simulink model "part2"  (R2020a)
settings: Solver=FixedStepAuto  StartTime=0.0  StopTime=150  FixedStep=0.1  RelTol=1e-3
values from neighbouring files (symbols this model uses):
  A = [zeros(3), eye(3) ... (first row only)    [initEKF.m]    (also in initEKF.mat = [0 0 0 -0.394784176044 0 0 0 0 0 0 -0.394784176044 0 ... (36)
  B = [0 0 0 0 0 0 1.46677031844e-07 0 0 0 0 0 ... (27 elements, 9x3)]    [ExtendedKalmanFilter.mat]    (also in initEKF.m = [zeros(6,3); initEKF.mat = [0 0 0 0 0 0 0 0 0 0 0 0 ... (45 elements, 15x3)]; initObserverInput.m = [zeros(6,3);zeros(3,3);zeros(3,3);invM]; initObserverInput.mat = [0 0 0 0 0 0 0 0 0 0 0 0 ... (45 elements, 15x3)])
  ConstSPSuge = 0    [ExtendedKalmanFilter.mat]    (also in doSimPart2.m; init.m; init1.m; init_weather.m)
  ConstSPSway = 0    [ExtendedKalmanFilter.mat]    (also in doSimPart2.m; init.m; init1.m; init_weather.m)
  ConstSPYaw = 0    [ExtendedKalmanFilter.mat]    (also in doSimPart2.m; init.m; init1.m; init_weather.m)
  Curent_Slaw_var = 0    [ExtendedKalmanFilter.mat]    (also in doSimPart2.m; init.m; init1.m; init_weather.m = 1)
  Current_Head_mu = 0.001    [ExtendedKalmanFilter.mat]    (also in doSimPart2.m; init.m; init1.m; init_weather.m)
  Current_Head_Sample_time = 1    [ExtendedKalmanFilter.mat]    (also in doSimPart2.m; init.m; init1.m; init_weather.m)
  Current_input_type = 0    [ExtendedKalmanFilter.mat]    (also in doSimPart2.m; init.m; init1.m; init_weather.m)
  Current_Speed = 0    [ExtendedKalmanFilter.mat]    (also in doSimPart2.m = 0.2; init.m; init1.m; init_weather.m = 0.2)
  CurrHead =     [ExtendedKalmanFilter.mat]
  D = [264860  0  0; 0  881640  0; 0  0  337740000]    [ExtendedKalmanFilter.mat]    (also in initEKF.m = [2.6486e5, 0, 0; initEKF.mat; initObserverInput.m = diag([2.6486e5, 8.8164e5, 3.3774e8]); initObserverInput.mat)
  E = [0 0 0 1 0 0 0 0 0 0 0 0 ... (27 elements, 9x3)]    [ExtendedKalmanFilter.mat]    (also in initEKF.m = [Ew, zeros(6,3); initEKF.mat = [0 0 0 0.01 0 0 0 0 0 0 0 0 ... (90 elements, 15x6)]; initObserverInput.m = [Ew, zeros(6,3); zeros(3), zeros(3); zeros(3), Eb; zeros(3),; initObserverInput.mat = [0 0 0 0.01 0 0 0 0 0 0 0 0 ... (90 elements, 15x6)])
  H = [1 0 0 0 1 0 0 0 1 0 0 0 ... (27 elements, 3x9)]    [ExtendedKalmanFilter.mat]    (also in initEKF.m = [C, eye(3), zeros(3), zeros(3)]; initEKF.mat = [0 0 0 0 0 0 0 0 0 1 0 0 ... (45 elements, 3x15)]; initObserverInput.m = [Cw, eye(3), zeros(3), zeros(3)]; initObserverInput.mat = [0 0 0 0 0 0 0 0 0 1 0 0 ... (45 elements, 3x15)])
  h = polar(Wind_Headind_EF.Data(:,1),Wind_Speed.Data(:,1))    [init.m]    (also in init1.m; initEKF.m = 0.1; initEKF.mat = 0.1; initObserverInput.m = 0.1)
  invM = inv(M)    [initEKF.m]    (also in initEKF.mat = [1.46677031844e-07  0  0; 0  1.2695973473e-07  9.23036390732; initObserverInput.m; initObserverInput.mat = [1.46677031844e-07  0  0; 0  1.2695973473e-07  9.23036390732)
  invT = inv(T)    [initEKF.m]    (also in initEKF.mat = [0.001  0  0; 0  0.001  0; 0  0  0.001])
  Kd_surge = 1868784.40925    [ExtendedKalmanFilter.mat]    (also in doSimPart2.m = 2*0.7*sqrt(6.4794^5+6.362*10^6)*sqrt(Kp_surge); init.m = 2*0.7*sqrt(6.4794^5+6.362*10^6)*sqrt(Kp_surge); init1.m = 2*0.7*sqrt(6.4794^5+6.362*10^6)*sqrt(Kp_surge); init_weather.m = 2*0.7*sqrt(6.4794^5+6.362*10^6)*sqrt(Kp_surge))
  Kd_sway = 3746851.89423    [ExtendedKalmanFilter.mat]    (also in doSimPart2.m = 2*0.7*sqrt(2.157*10^6+6.362*10^6)*sqrt(Kp_sway); init.m = 2*0.7*sqrt(2.157*10^6+6.362*10^6)*sqrt(Kp_sway); init1.m = 2*0.7*sqrt(2.157*10^6+6.362*10^6)*sqrt(Kp_sway); init_weather.m = 2*0.7*sqrt(2.157*10^6+6.362*10^6)*sqrt(Kp_sway))
  Kd_yaw = 3338344318.3    [ExtendedKalmanFilter.mat]    (also in doSimPart2.m = 2*0.7*sqrt(1.0711*10^9+2.724*10^9)*sqrt(Kp_yaw); init.m = 2*0.7*sqrt(1.0711*10^9+2.724*10^9)*sqrt(Kp_yaw); init1.m = 2*0.7*sqrt(1.0711*10^9+2.724*10^9)*sqrt(Kp_yaw); init_weather.m = 2*0.7*sqrt(1.0711*10^9+2.724*10^9)*sqrt(Kp_yaw))
  Ki_surge = 18000    [ExtendedKalmanFilter.mat]    (also in doSimPart2.m; init.m; init1.m; init_weather.m)
  Ki_sway = 80000    [ExtendedKalmanFilter.mat]    (also in doSimPart2.m; init.m; init1.m; init_weather.m)
  Ki_yaw = 150000000    [ExtendedKalmanFilter.mat]    (also in doSimPart2.m; init.m; init1.m; init_weather.m = 150000)
  Kp_surge = 279569.493868    [ExtendedKalmanFilter.mat]    (also in doSimPart2.m; init.m; init1.m; init_weather.m = 195698.645708)
  Kp_sway = 840791.598929    [ExtendedKalmanFilter.mat]    (also in doSimPart2.m; init.m; init1.m; init_weather.m = 588554.11925)
  Kp_yaw = 1498245426.5    [ExtendedKalmanFilter.mat]    (also in doSimPart2.m; init.m; init1.m; init_weather.m = 104877179.855)
  p_bar = zeros(15)    [initEKF.m]    (also in initEKF.mat = [0 0 0 0 0 0 0 0 0 0 0 0 ... (225 elements, 15x15)])
  Q = [1000000000000  0  0; 0  1000000000000  0; 0  0  100000000000000]    [ExtendedKalmanFilter.mat]    (also in initEKF.m = [10^4, 0, 0, 0, 0, 0; initEKF.mat = [10000 0 0 0 0 0 0 10000 0 0 0 0 ... (36 elements, 6x6)]; initObserverInput.m = diag([ 10^4 10^4 10^3 10^9 10^9 10^9]); initObserverInput.mat = [10000 0 0 0 0 0 0 10000 0 0 0 0 ... (36 elements, 6x6)])
  R = [1.15e-05  0  0; 0  1.2e-06  0; 0  0  4e-08]    [ExtendedKalmanFilter.mat]    (also in initEKF.m = [1, 0,0; initEKF.mat = [1  0  0; 0  1  0; 0  0  0.1]; initObserverInput.m = diag([1,1,0.1]); initObserverInput.mat = [1  0  0; 0  1  0; 0  0  0.1])
  thrusters =     [ExtendedKalmanFilter.mat]
  typeOfSimulation = 2    [ExtendedKalmanFilter.mat]    (also in doSimPart2.m = 0; init.m; init1.m; init_weather.m)
  vessel =     [ExtendedKalmanFilter.mat]
  Wind_gust_k = 0.0026    [ExtendedKalmanFilter.mat]    (also in doSimPart2.m; init.m; init1.m; init_weather.m)
  Wind_gust_L = 1800    [ExtendedKalmanFilter.mat]    (also in doSimPart2.m; init.m; init1.m; init_weather.m)
  Wind_gust_nfreq = 1000    [ExtendedKalmanFilter.mat]    (also in doSimPart2.m; init.m; init1.m; init_weather.m)
  Wind_gust_phi = [1.94720348827 2.24175439974 2.07841268688 2.94269508899 2.5189968857 3.92559282604 1.02965824361 5.79326836705 3.39416152385 6.24100933894 1.9296881265 4.15801677987 ... (1000 elements, 1000x1)]    [ExtendedKalmanFilter.mat]    (also in doSimPart2.m = 2*pi * rand(Wind_gust_nfreq,1); init.m = 2*pi * rand(Wind_gust_nfreq,1); init1.m = 2*pi * rand(Wind_gust_nfreq,1); init_weather.m = 2*pi * rand(Wind_gust_nfreq,1))
  Wind_Gust_type = 0    [ExtendedKalmanFilter.mat]    (also in doSimPart2.m = 1; init.m; init1.m; init_weather.m = 1)
  Wind_Head_mean = 1.57079632679    [ExtendedKalmanFilter.mat]    (also in doSimPart2.m = vector_Headings_rad; init.m; init1.m; init_weather.m = 0)
  Wind_Head_mu = 0.001    [ExtendedKalmanFilter.mat]    (also in doSimPart2.m; init.m; init1.m; init_weather.m)
  Wind_Head_Sample_time = 1    [ExtendedKalmanFilter.mat]    (also in doSimPart2.m; init.m; init1.m; init_weather.m)
  Wind_Heading_type = 0    [ExtendedKalmanFilter.mat]    (also in doSimPart2.m; init.m; init1.m; init_weather.m = 1)
  Wind_U10 = 0    [ExtendedKalmanFilter.mat]    (also in doSimPart2.m = 15; init.m; init1.m; init_weather.m)
  Wind_U_mean = 0    [ExtendedKalmanFilter.mat]    (also in doSimPart2.m = Umean; init.m = Umean; init1.m = Umean; init_weather.m = Umean)
  Wind_U_mu = 0.001    [ExtendedKalmanFilter.mat]    (also in doSimPart2.m; init.m; init1.m; init_weather.m)
  Wind_U_Sample_time = 1    [ExtendedKalmanFilter.mat]    (also in doSimPart2.m; init.m; init1.m; init_weather.m)
  Wind_U_type = 0    [ExtendedKalmanFilter.mat]    (also in doSimPart2.m = 1; init.m; init1.m; init_weather.m = 1)
  x_bar = zeros(15,1)    [initEKF.m]    (also in initEKF.mat = [0 0 0 0 0 0 0 0 0 0 0 0 ... (15 elements, 15x1)])
undefined symbols (not defined in the file or in its folder): Hoerner
libraries: marine_gnc x10, simulink x4, marine_hydro x2
(part 1 of 2)
settings Model: Creator=jonbjor  LastModifiedBy=maria
settings DataIOCC: ReturnWorkspaceOutputs=off
settings DebuggingCC: ArithmeticOperatorsInVariantConditions=warning
settings SFSimCC: SimUseLocalCustomCode=off  CustomCodeUndefinedFunction=UseInterfaceOnly
settings RTWCC: RTWUseLocalCustomCode=off

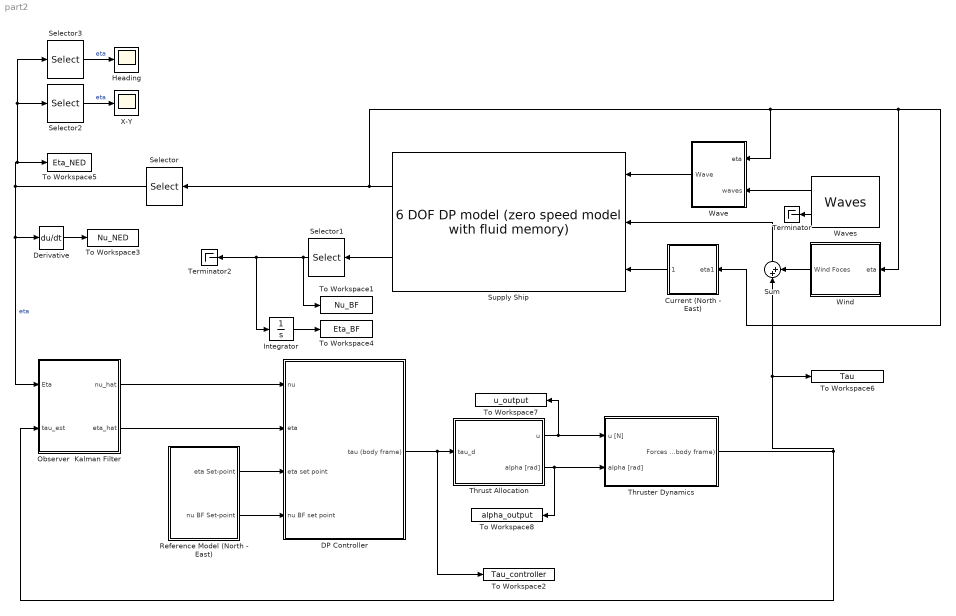
== system part2 ==
  Current (North - East) : Subsystem
  DP Controller : Subsystem
  Derivative : Derivative
  Heading : Scope
  Integrator : Integrator
  Observer  Kalman Filter : Subsystem
  Reference Model (North - East) : Subsystem
  Selector : Selector  InputPortWidth=6  IndexOptions=Index vector (dialog)  Indices=[1 2 6]  OutputSizes=1
  Selector1 : Selector  InputPortWidth=6  IndexOptions=Index vector (dialog)  Indices=[1 2 6]  OutputSizes=1
  Selector2 : Selector  InputPortWidth=3  IndexOptions=Index vector (dialog)  Indices=[1 2]  OutputSizes=1
  Selector3 : Selector  InputPortWidth=3  IndexOptions=Index vector (dialog)  Indices=3  OutputSizes=1
  Sum : Sum  Inputs=|++
  Supply Ship : marine_hydro/Hydro Library/6 DOF DP model  (zero speed model with fluid memory)  ABC=vesselABC  rho=1025  Axc=0.9*vessel.main.T*vessel.main.B  Ayc=0.9*vessel.main.T*vessel.main.Lpp  CX=1  CY_2D=Hoerner(vessel.main.B,vessel.main.T)  Bv=vessel.Bv  mask(6 DOF zero speed model){}
      link override "Integrator1 ": InitialCondition=nu0
      link override Integrator2: InitialCondition=eta0
      settings: SourceProductName=MSS Hydro
      mask Display:
      | image('supply.jpg');
      | color('white'); port_label('output', 1, 'eta')
      | color('white'); port_label('output', 2, 'nu')
      | color('white'); port_label('input', 1, 'tau_wave')
      | color('white'); port_label('input', 2, 'tau')
      | color('white'); port_label('input', 3, 'nu_c')
  Terminator : Terminator
  Terminator2 : Terminator
  Thrust Allocation : Subsystem
  Thruster Dynamics : Subsystem  mask{thrusterfault=off}
      mask prompts: thrusterfault "Fault on thruster #2 and #5?"
  To Workspace1 : ToWorkspace  VariableName=Nu_BF  SaveFormat=Timeseries  SampleTime=-1
  To Workspace2 : ToWorkspace  VariableName=Tau_controller  SaveFormat=Timeseries  SampleTime=-1
  To Workspace3 : ToWorkspace  VariableName=Nu_NED  SaveFormat=Timeseries  SampleTime=-1
  To Workspace4 : ToWorkspace  VariableName=Eta_BF  SaveFormat=Timeseries  SampleTime=-1
  To Workspace5 : ToWorkspace  VariableName=Eta_NED  SaveFormat=Timeseries  SampleTime=-1
  To Workspace6 : ToWorkspace  VariableName=Tau  SaveFormat=Timeseries  SampleTime=-1
  To Workspace7 : ToWorkspace  VariableName=u_output  SaveFormat=Timeseries  SampleTime=-1
  To Workspace8 : ToWorkspace  VariableName=alpha_output  SaveFormat=Timeseries  SampleTime=-1
  Wave : Subsystem  mask{waveforces=on}
      mask prompts: waveforces "Waveforces enabled"
  Waves : marine_gnc/Environment/Waves/Waves  spectrum_type=ITTC  disp_flag=on  plot_spectrum=off  plot_realization=off  hs=Significant_wave_height_Hs  omega_peak=Peak_frequency_omega_0  psi_mean=Mean_wave_direction  gamma=-1  spread=2  depth=inf  nfreq=20  ndir=10  energylim=0.005  freq_cutoff=3  dir_cutoff=0  rand_seed=123  rand_freq=on  rand_dir=on  Zeta_a=0  Omega=0  Phase=0  Wavenum=0  Psi=0
      settings: SourceProductName=MSS GNC
  Wind : Subsystem
  X-Y : Scope
  wires:
  Supply Ship/2 -> Selector1/1
  Reference Model (North - East)/1(eta Set-point) -> DP Controller/3(eta set point)
  Supply Ship/1 -> Current (North - East)/1(eta1), Wind/1(eta), Wave/1(eta), Selector/1
  Waves/1 -> Wave/2(waves)
  Waves/2 -> Terminator/1
  Sum/1 -> Supply Ship/2
  Thrust Allocation/2(alpha [rad]) -> Thruster Dynamics/2(alpha [rad]), To Workspace8/1
  Current (North - East)/1(Current) -> Supply Ship/3
  Selector/1 -> Observer  Kalman Filter/1(Eta), Derivative/1, Selector3/1, Selector2/1, To Workspace5/1  "eta"
  Wind/1(Wind Foces) -> Sum/2
  Derivative/1 -> To Workspace3/1
  Integrator/1 -> To Workspace4/1
  Wave/1(Wave) -> Supply Ship/1
  Reference Model (North - East)/2(nu BF Set-point) -> DP Controller/4(nu BF set point)
  Thrust Allocation/1(u) -> Thruster Dynamics/1(u [N]), To Workspace7/1
  Selector1/1 -> To Workspace1/1, Terminator2/1, Integrator/1
  Observer  Kalman Filter/1(nu_hat) -> DP Controller/1(nu)
  Observer  Kalman Filter/2(eta_hat) -> DP Controller/2(eta)
  Selector2/1 -> X-Y/1  "eta"
  Selector3/1 -> Heading/1  "eta"
  DP Controller/1(tau (body frame)) -> To Workspace2/1, Thrust Allocation/1(tau_d)
  Thruster Dynamics/1("Forces (body frame) ") -> Observer  Kalman Filter/2(tau_est), Sum/1, To Workspace6/1

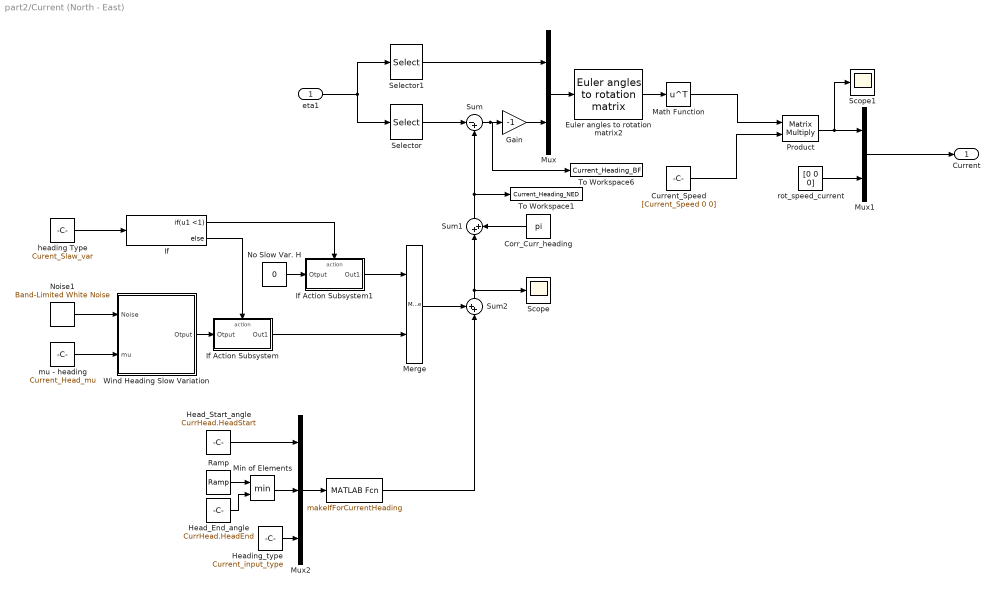
== system part2/Current (North - East) ==
  eta1 : Inport
  " " : MATLABFcn  MATLABFcn=makeIfForCurrentHeading
  Corr_Curr_heading : Constant  Value=pi
  Current_Speed : Constant  Value=[Current_Speed 0 0]
  Euler angles to rotation matrix2 : marine_gnc/Models/ Kinematics/Euler angles to rotation matrix
      settings: SourceProductName=MSS GNC
  Gain : Gain  Gain=-1
  Head_End_angle : Constant  Value=CurrHead.HeadEnd
  Head_Start_angle : Constant  Value=CurrHead.HeadStart
  Heading_type : Constant  Value=Current_input_type
  If : If  IfExpression=u1 <1
  If Action Subsystem : Subsystem  TreatAsAtomicUnit=on
  If Action Subsystem1 : Subsystem  TreatAsAtomicUnit=on
  Math Function : Math  Operator=transpose  SaturateOnIntegerOverflow=on
  Merge : Merge
  Min of Elements : MinMax  Inputs=2
  Mux : Mux  Inputs=2
  Mux1 : Mux  Inputs=2
  Mux2 : Mux  Inputs=3
  No Slow Var. H : Constant  Value=0
  Noise1 : simulink/Sources/Band-Limited White Noise  Cov=Current_Head_noise_power  Ts=Current_Head_Sample_time  seed=Current_Head_Seed
  Product : Product  Inputs=**  Multiplication=Matrix(*)  SaturateOnIntegerOverflow=on  OutDataTypeStr=Inherit: Same as first input
  Ramp : simulink/Sources/Ramp  slope=CurrHead.Slope  start=CurrHead.TimeStart  InitialOutput=CurrHead.HeadStart
  Scope : Scope
  Scope1 : Scope
  Selector : Selector  InputPortWidth=6  IndexOptions=Index vector (dialog)  Indices=[6]  OutputSizes=1
  Selector1 : Selector  InputPortWidth=6  IndexOptions=Index vector (dialog)  Indices=[4 5]  OutputSizes=1
  Sum : Sum  Inputs=|-+
  Sum1 : Sum  Inputs=|++
  Sum2 : Sum  Inputs=++|
  To Workspace1 : ToWorkspace  VariableName=Current_Heading_NED  SaveFormat=Timeseries  SampleTime=-1
  To Workspace6 : ToWorkspace  VariableName=Current_Heading_BF  SaveFormat=Timeseries  SampleTime=-1
  Wind Heading Slow Variation : Subsystem
  heading Type : Constant  Value=Curent_Slaw_var
  mu - heading : Constant  Value=Current_Head_mu
  rot_speed_current : Constant  Value=[0 0 0]
  Current : Outport  VectorParamsAs1DForOutWhenUnconnected=off
  wires:
  Sum2/1 -> Scope/1, Sum1/1
  eta1/1 -> Selector/1, Selector1/1
  Merge/1 -> Sum2/1
  mu - heading/1 -> Wind Heading Slow Variation/2(mu)
  " "/1 -> Sum2/2
  If Action Subsystem1/1(Out1) -> Merge/1
  Sum1/1 -> To Workspace1/1, Sum/2
  If Action Subsystem/1(Out1) -> Merge/2
  Wind Heading Slow Variation/1(Otput) -> If Action Subsystem/1(Otput)
  No Slow Var. H/1 -> If Action Subsystem1/1(Otput)
  If/2 -> If Action Subsystem/Action
  Selector1/1 -> Mux/1
  If/1 -> If Action Subsystem1/Action
  Selector/1 -> Sum/1
  Mux/1 -> Euler angles to rotation matrix2/1
  heading Type/1 -> If/1
  Corr_Curr_heading/1 -> Sum1/2
  Product/1 -> Scope1/1, Mux1/1
  Noise1/1 -> Wind Heading Slow Variation/1(Noise)
  Current_Speed/1 -> Product/2
  Head_Start_angle/1 -> Mux2/1
  Euler angles to rotation matrix2/1 -> Math Function/1
  rot_speed_current/1 -> Mux1/2
  Mux2/1 -> " "/1
  Mux1/1 -> Current/1
  Min of Elements/1 -> Mux2/2
  Math Function/1 -> Product/1
  Heading_type/1 -> Mux2/3
  Ramp/1 -> Min of Elements/1
  Head_End_angle/1 -> Min of Elements/2
  Sum/1 -> Gain/1, To Workspace6/1
  Gain/1 -> Mux/2

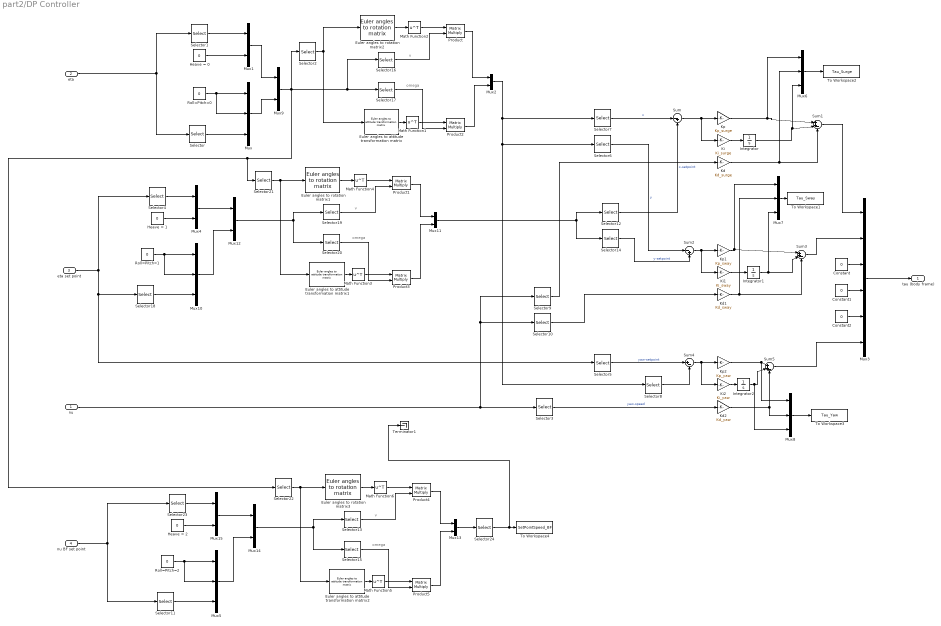
== system part2/DP Controller ==
  note: omega
  note: omega
  note: v
  note: v
  note: omega
  note: v
  nu : Inport
  eta : Inport  Port=2
  eta set point : Inport  Port=3
  nu BF set point : Inport  Port=4
  Constant : Constant  Value=0
  Constant1 : Constant  Value=0
  Constant2 : Constant  Value=0
  Euler angles to rotation matrix1 : marine_gnc/Models/ Kinematics/Euler angles to rotation matrix
      settings: SourceProductName=MSS GNC
  Euler angles to rotation matrix2 : marine_gnc/Models/ Kinematics/Euler angles to rotation matrix
      settings: SourceProductName=MSS GNC
  Euler angles to rotation matrix3 : marine_gnc/Models/ Kinematics/Euler angles to rotation matrix
      settings: SourceProductName=MSS GNC
  Euler angles to attitude transformation matrix : marine_gnc/Models/ Kinematics/Euler angles to attitude transformation matrix
      settings: SourceProductName=MSS GNC
  Euler angles to attitude transformation matrix1 : marine_gnc/Models/ Kinematics/Euler angles to attitude transformation matrix
      settings: SourceProductName=MSS GNC
  Euler angles to attitude transformation matrix2 : marine_gnc/Models/ Kinematics/Euler angles to attitude transformation matrix
      settings: SourceProductName=MSS GNC
  Heave = 0 : Constant  Value=0
  Heave = 1 : Constant  Value=0
  Heave = 2 : Constant  Value=0
  Integrator : Integrator
  Integrator1 : Integrator
  Integrator2 : Integrator
  Kd : Gain  Gain=Kd_surge
  Kd1 : Gain  Gain=Kd_sway
  Kd2 : Gain  Gain=Kd_yaw
  Ki : Gain  Gain=Ki_surge
  Ki1 : Gain  Gain=Ki_sway
  Ki2 : Gain  Gain=Ki_yaw
  Kp : Gain  Gain=Kp_surge
  Kp1 : Gain  Gain=Kp_sway
  Kp2 : Gain  Gain=Kp_yaw
  Math Function{1..6} (6 alike) : Math  Operator=transpose  SaturateOnIntegerOverflow=on
  Mux{,5..8,10} (6 alike) : Mux  Inputs=3
  Mux{1..2,4,9,11..15} (9 alike) : Mux  Inputs=2
  Mux3 : Mux  Inputs=6
  Product{,1..5} (6 alike) : Product  Inputs=**  Multiplication=Matrix(*)  SaturateOnIntegerOverflow=on  OutDataTypeStr=Inherit: Same as first input
  Roll=Pitch=0 : Constant  Value=0
  Roll=Pitch=1 : Constant  Value=0
  Roll=Pitch=2 : Constant  Value=0
  Selector{,5,11,18} (4 alike) : Selector  InputPortWidth=3  IndexOptions=Index vector (dialog)  Indices=[3]  OutputSizes=1
  Selector1 : Selector  InputPortWidth=3  IndexOptions=Index vector (dialog)  Indices=[1 2]  OutputSizes=1
  Selector10 : Selector  InputPortWidth=3  IndexOptions=Index vector (dialog)  Indices=2  OutputSizes=1
  Selector12 : Selector  InputPortWidth=6  IndexOptions=Index vector (dialog)  Indices=1  OutputSizes=1
  Selector13 : Selector  InputPortWidth=6  IndexOptions=Index vector (dialog)  Indices=[1 2 3]  OutputSizes=1
  Selector14 : Selector  InputPortWidth=6  IndexOptions=Index vector (dialog)  Indices=2  OutputSizes=1
  Selector{2,15,17,20..22} (6 alike) : Selector  InputPortWidth=6  IndexOptions=Index vector (dialog)  Indices=[4 5 6]  OutputSizes=1
  Selector16 : Selector  InputPortWidth=6  IndexOptions=Index vector (dialog)  Indices=[1 2 3]  OutputSizes=1
  Selector19 : Selector  InputPortWidth=6  IndexOptions=Index vector (dialog)  Indices=[1 2 3]  OutputSizes=1
  Selector23 : Selector  InputPortWidth=3  IndexOptions=Index vector (dialog)  Indices=[1 2]  OutputSizes=1
  Selector24 : Selector  InputPortWidth=6  IndexOptions=Index vector (dialog)  Indices=[1 2 6]  OutputSizes=1
  Selector3 : Selector  InputPortWidth=3  IndexOptions=Index vector (dialog)  Indices=3  OutputSizes=1
  Selector4 : Selector  InputPortWidth=3  IndexOptions=Index vector (dialog)  Indices=[1 2]  OutputSizes=1
  Selector6 : Selector  InputPortWidth=6  IndexOptions=Index vector (dialog)  Indices=2  OutputSizes=1
  Selector7 : Selector  InputPortWidth=6  IndexOptions=Index vector (dialog)  Indices=1  OutputSizes=1
  Selector8 : Selector  InputPortWidth=6  IndexOptions=Index vector (dialog)  Indices=[6]  OutputSizes=1
  Selector9 : Selector  InputPortWidth=3  IndexOptions=Index vector (dialog)  Indices=1  OutputSizes=1
  Sum : Sum  Inputs=|-+
  Sum1 : Sum  Inputs=|++-
  Sum2 : Sum  Inputs=|-+
  Sum3 : Sum  Inputs=|++-
  Sum4 : Sum  Inputs=|+-
  Sum5 : Sum  Inputs=|++-
  Terminator1 : Terminator
  To Workspace1 : ToWorkspace  VariableName=Tau_Sway  SaveFormat=Timeseries  SampleTime=-1
  To Workspace2 : ToWorkspace  VariableName=Tau_Surge  SaveFormat=Timeseries  SampleTime=-1
  To Workspace3 : ToWorkspace  VariableName=Tau_Yaw  SaveFormat=Timeseries  SampleTime=-1
  To Workspace4 : ToWorkspace  VariableName=SetPointSpeed_BF  SaveFormat=Timeseries  SampleTime=-1
  tau (body frame) : Outport  VectorParamsAs1DForOutWhenUnconnected=off
  wires:
  Selector20/1 -> Product3/2
  Mux4/1 -> Mux12/1
  Selector2/1 -> Euler angles to attitude transformation matrix/1, Euler angles to rotation matrix2/1
  Product1/1 -> Mux11/1
  Mux10/1 -> Mux12/2
  Mux8/1 -> To Workspace3/1
  Euler angles to rotation matrix1/1 -> Math Function4/1
  Product/1 -> Mux2/1
  Selector17/1 -> Product2/2
  Kp2/1 -> Mux8/1, Sum5/1
  Ki1/1 -> Integrator1/1
  Mux6/1 -> To Workspace2/1
  Euler angles to rotation matrix2/1 -> Math Function2/1
  Selector6/1 -> Sum2/1  "y"
  Selector/1 -> Mux/3
  Sum4/1 -> Ki2/1, Kp2/1
  Kp1/1 -> Mux7/1, Sum3/1
  Product2/1 -> Mux2/2
  Constant1/1 -> Mux3/4
  Selector18/1 -> Mux10/3
  Sum2/1 -> Ki1/1, Kp1/1
  eta set point/1 -> Selector4/1, Selector18/1, Selector5/1
  Kd1/1 -> Mux7/2, Sum3/3
  Mux1/1 -> Mux9/1
  Sum1/1 -> Mux3/1
  Kd2/1 -> Mux8/2, Sum5/3
  Roll=Pitch=1/1 -> Mux10/1, Mux10/2
  Ki/1 -> Integrator/1
  Product3/1 -> Mux11/2
  Selector4/1 -> Mux4/1
  Math Function4/1 -> Product1/1
  Selector1/1 -> Mux1/1
  Selector12/1 -> Sum/2  "x-setpoint"
  Math Function1/1 -> Product2/1
  Selector5/1 -> Sum4/1  "yaw-setpoint"
  Mux7/1 -> To Workspace1/1
  Selector3/1 -> Kd2/1  "yaw-speed"
  Roll=Pitch=0/1 -> Mux/1, Mux/2
  Selector8/1 -> Sum4/2
  Selector10/1 -> Kd1/1
  Constant/1 -> Mux3/3
  Math Function3/1 -> Product3/1
  Constant2/1 -> Mux3/5
  Mux/1 -> Mux9/2
  eta/1 -> Selector/1, Selector1/1
  Sum5/1 -> Mux3/6
  Mux3/1 -> tau (body frame)/1
  Integrator2/1 -> Mux8/3, Sum5/2
  Selector9/1 -> Kd/1
  Euler angles to attitude transformation matrix/1 -> Math Function1/1
  Selector19/1 -> Product1/2
  Mux11/1 -> Selector14/1, Selector12/1
  Integrator1/1 -> Sum3/2, Mux7/3
  Heave = 1/1 -> Mux4/2
  Selector16/1 -> Product/2
  Euler angles to attitude transformation matrix1/1 -> Math Function3/1
  Heave = 0/1 -> Mux1/2
  Integrator/1 -> Mux6/3, Sum1/2
  Kd/1 -> Mux6/2, Sum1/3
  Mux2/1 -> Selector6/1, Selector8/1, Selector7/1
  Selector14/1 -> Sum2/2  "y-setpoint"
  Selector21/1 -> Euler angles to rotation matrix1/1, Euler angles to attitude transformation matrix1/1
  Ki2/1 -> Integrator2/1
  Mux12/1 -> Selector20/1, Selector19/1
  Sum/1 -> Ki/1, Kp/1
  Math Function2/1 -> Product/1
  Kp/1 -> Mux6/1, Sum1/1
  Selector7/1 -> Sum/1  "x"
  Sum3/1 -> Mux3/2
  nu/1 -> Selector9/1, Selector10/1, Selector3/1
  Selector15/1 -> Product5/2
  Selector23/1 -> Mux15/1
  Selector22/1 -> Euler angles to rotation matrix3/1, Euler angles to attitude transformation matrix2/1
  Mux14/1 -> Selector15/1, Selector13/1
  Mux9/1 -> Selector21/1, Selector22/1, Selector2/1, Selector17/1, Selector16/1
  Math Function5/1 -> Product5/1
  Heave = 2/1 -> Mux15/2
  Euler angles to attitude transformation matrix2/1 -> Math Function5/1
  Selector13/1 -> Product4/2
  Product5/1 -> Mux13/2
  Roll=Pitch=2/1 -> Mux5/1, Mux5/2
  nu BF set point/1 -> Selector23/1, Selector11/1
  Selector11/1 -> Mux5/3
  Euler angles to rotation matrix3/1 -> Math Function6/1
  Mux5/1 -> Mux14/2
  Math Function6/1 -> Product4/1
  Mux15/1 -> Mux14/1
  Product4/1 -> Mux13/1
  Mux13/1 -> Selector24/1
  Selector24/1 -> To Workspace4/1, Terminator1/1

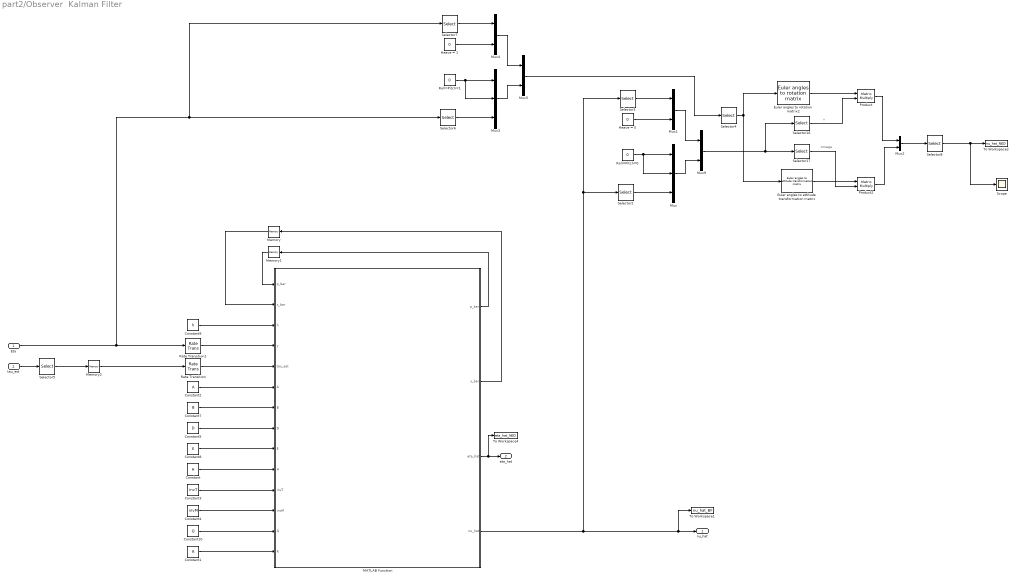
== system part2/Observer  Kalman Filter ==
  note: omega
  note: v
  Eta : Inport
  tau_est : Inport  Port=2
  Constant : Constant  Value=H
  Constant1 : Constant  Value=R
  Constant10 : Constant  Value=Q
  Constant2 : Constant  Value=A
  Constant3 : Constant  Value=invT
  Constant4 : Constant  Value=invM
  Constant5 : Constant  Value=D
  Constant7 : Constant  Value=B
  Constant8 : Constant  Value=E
  Constant9 : Constant  Value=h
  Euler angles to rotation matrix2 : marine_gnc/Models/ Kinematics/Euler angles to rotation matrix
      settings: SourceProductName=MSS GNC
  Euler angles to attitude transformation matrix : marine_gnc/Models/ Kinematics/Euler angles to attitude transformation matrix
      settings: SourceProductName=MSS GNC
  Heave = 0 : Constant  Value=0
  Heave = 1 : Constant  Value=0
  MATLAB Function : MATLAB Function  TreatAsAtomicUnit=on
  Memory : Memory  InitialCondition=x_bar  InheritSampleTime=on  LinearizeMemory=on  LinearizeAsDelay=on
  Memory1 : Memory  InitialCondition=p_bar  InheritSampleTime=on  LinearizeMemory=on  LinearizeAsDelay=on
  Memory2 : Memory  InheritSampleTime=on
  Mux : Mux  Inputs=3
  Mux{1..2,4..5,9} (5 alike) : Mux  Inputs=2
  Mux3 : Mux  Inputs=3
  Product : Product  Inputs=**  Multiplication=Matrix(*)  SaturateOnIntegerOverflow=on  OutDataTypeStr=Inherit: Same as first input
  Product2 : Product  Inputs=**  Multiplication=Matrix(*)  SaturateOnIntegerOverflow=on  OutDataTypeStr=Inherit: Same as first input
  Rate Transition : RateTransition  OutPortSampleTime=h
  Rate Transition1 : RateTransition  OutPortSampleTime=h
  Roll=Pitch=0 : Constant  Value=0
  Roll=Pitch=1 : Constant  Value=0
  Scope : Scope
  Selector16 : Selector  InputPortWidth=6  IndexOptions=Index vector (dialog)  Indices=[1 2 3]  OutputSizes=1
  Selector17 : Selector  InputPortWidth=6  IndexOptions=Index vector (dialog)  Indices=[4 5 6]  OutputSizes=1
  Selector2 : Selector  InputPortWidth=3  IndexOptions=Index vector (dialog)  Indices=[3]  OutputSizes=1
  Selector3 : Selector  InputPortWidth=3  IndexOptions=Index vector (dialog)  Indices=[1 2]  OutputSizes=1
  Selector4 : Selector  InputPortWidth=6  IndexOptions=Index vector (dialog)  Indices=[4 5 6]  OutputSizes=1
  Selector5 : Selector  InputPortWidth=6  IndexOptions=Index vector (dialog)  Indices=[1 2 6]  OutputSizes=1
  Selector6 : Selector  InputPortWidth=3  IndexOptions=Index vector (dialog)  Indices=[3]  OutputSizes=1
  Selector7 : Selector  InputPortWidth=3  IndexOptions=Index vector (dialog)  Indices=[1 2]  OutputSizes=1
  Selector8 : Selector  InputPortWidth=6  IndexOptions=Index vector (dialog)  Indices=[1 2 6]  OutputSizes=1
  To Workspace1 : ToWorkspace  VariableName=nu_hat_BF  SaveFormat=Timeseries  SampleTime=-1
  To Workspace2 : ToWorkspace  VariableName=nu_hat_NED  SaveFormat=Timeseries  SampleTime=-1
  To Workspace4 : ToWorkspace  VariableName=eta_hat_NED  SaveFormat=Timeseries  SampleTime=-1
  nu_hat : Outport  VectorParamsAs1DForOutWhenUnconnected=off
  eta_hat : Outport  Port=2  VectorParamsAs1DForOutWhenUnconnected=off
  wires:
  Selector5/1 -> Memory2/1
  Memory2/1 -> Rate Transition/1
  tau_est/1 -> Selector5/1
  Product2/1 -> Mux2/2
  Selector17/1 -> Product2/2
  Selector4/1 -> Euler angles to attitude transformation matrix/1, Euler angles to rotation matrix2/1
  Selector16/1 -> Product/2
  Roll=Pitch=0/1 -> Mux/1, Mux/2
  MATLAB Function/4(nu_hat) -> Selector3/1, Selector2/1, To Workspace1/1, nu_hat/1
  Product/1 -> Mux2/1
  Mux9/1 -> Selector17/1, Selector16/1
  Selector2/1 -> Mux/3
  Mux/1 -> Mux9/2
  Euler angles to attitude transformation matrix/1 -> Product2/1
  Mux1/1 -> Mux9/1
  Euler angles to rotation matrix2/1 -> Product/1
  Heave = 0/1 -> Mux1/2
  Selector3/1 -> Mux1/1
  Mux5/1 -> Selector4/1
  Mux3/1 -> Mux5/2
  Roll=Pitch=1/1 -> Mux3/1, Mux3/2
  Selector7/1 -> Mux4/1
  Heave = 1/1 -> Mux4/2
  Selector6/1 -> Mux3/3
  Mux4/1 -> Mux5/1
  Mux2/1 -> Selector8/1
  Selector8/1 -> Scope/1, To Workspace2/1
  Constant8/1 -> MATLAB Function/9(E)
  Memory/1 -> MATLAB Function/2("x_bar ")
  Constant9/1 -> MATLAB Function/3(h)
  Constant/1 -> MATLAB Function/10(H)
  Constant3/1 -> MATLAB Function/11(invT)
  Constant5/1 -> MATLAB Function/8(D)
  Constant4/1 -> MATLAB Function/12(invM)
  Rate Transition/1 -> MATLAB Function/5(tau_est)
  MATLAB Function/3(eta_hat) -> To Workspace4/1, eta_hat/1
  Constant10/1 -> MATLAB Function/13(Q)
  Constant2/1 -> MATLAB Function/6(A)
  MATLAB Function/1(p_bar) -> Memory1/1
  MATLAB Function/2(x_bar) -> Memory/1
  Memory1/1 -> MATLAB Function/1("p_bar ")
  Constant7/1 -> MATLAB Function/7(B)
  Eta/1 -> Rate Transition1/1, Selector7/1, Selector6/1
  Rate Transition1/1 -> MATLAB Function/4(y)
  Constant1/1 -> MATLAB Function/14(R)

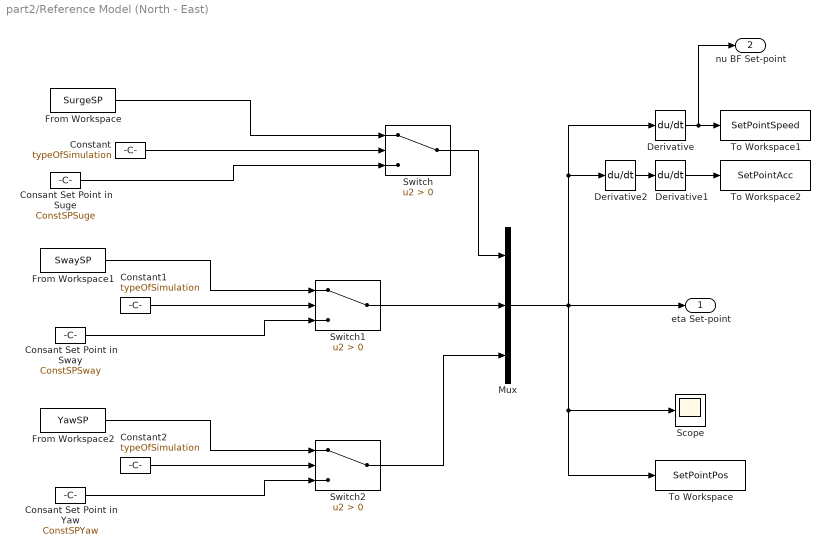
== system part2/Reference Model (North - East) ==
  Consant Set Point in Suge : Constant  Value=ConstSPSuge
  Consant Set Point in Sway : Constant  Value=ConstSPSway
  Consant Set Point in Yaw : Constant  Value=ConstSPYaw
  Constant : Constant  Value=typeOfSimulation
  Constant1 : Constant  Value=typeOfSimulation
  Constant2 : Constant  Value=typeOfSimulation
  Derivative : Derivative
  Derivative1 : Derivative
  Derivative2 : Derivative
  From Workspace : FromWorkspace  VariableName=SurgeSP
  From Workspace1 : FromWorkspace  VariableName=SwaySP
  From Workspace2 : FromWorkspace  VariableName=YawSP
  Mux : Mux  Inputs=3
  Scope : Scope
  Switch : Switch  Criteria=u2 > Threshold
  Switch1 : Switch  Criteria=u2 > Threshold
  Switch2 : Switch  Criteria=u2 > Threshold
  To Workspace : ToWorkspace  VariableName=SetPointPos  SaveFormat=Timeseries  SampleTime=-1
  To Workspace1 : ToWorkspace  VariableName=SetPointSpeed  SaveFormat=Timeseries  SampleTime=-1
  To Workspace2 : ToWorkspace  VariableName=SetPointAcc  SaveFormat=Timeseries  SampleTime=-1
  eta Set-point : Outport  VectorParamsAs1DForOutWhenUnconnected=off
  nu BF Set-point : Outport  Port=2  VectorParamsAs1DForOutWhenUnconnected=off
  wires:
  Derivative1/1 -> To Workspace2/1
  Constant1/1 -> Switch1/2
  Switch2/1 -> Mux/3
  From Workspace1/1 -> Switch1/1
  Constant2/1 -> Switch2/2
  Derivative2/1 -> Derivative1/1
  Constant/1 -> Switch/2
  Switch/1 -> Mux/1
  Consant Set Point in Suge/1 -> Switch/3
  Consant Set Point in Sway/1 -> Switch1/3
  From Workspace2/1 -> Switch2/1
  Switch1/1 -> Mux/2
  Consant Set Point in Yaw/1 -> Switch2/3
  Derivative/1 -> nu BF Set-point/1, To Workspace1/1
  From Workspace/1 -> Switch/1
  Mux/1 -> To Workspace/1, Scope/1, eta Set-point/1, Derivative2/1, Derivative/1

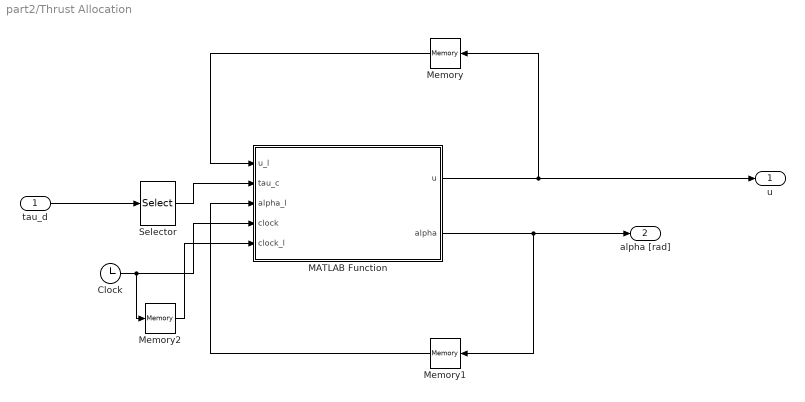
== system part2/Thrust Allocation ==
  tau_d : Inport
  Clock : Clock
  MATLAB Function : MATLAB Function  TreatAsAtomicUnit=on
  Memory : Memory  InitialCondition=[0 0 0 0 0]'
  Memory1 : Memory  InitialCondition=[0 0 0 0 0]'
  Memory2 : Memory
  Selector : Selector  InputPortWidth=6  IndexOptions=Index vector (dialog)  Indices=[1 2 6]  OutputSizes=1
  u : Outport  VectorParamsAs1DForOutWhenUnconnected=off
  alpha [rad] : Outport  Port=2  VectorParamsAs1DForOutWhenUnconnected=off
  wires:
  Selector/1 -> MATLAB Function/2(tau_c)
  Memory1/1 -> MATLAB Function/3(alpha_l)
  tau_d/1 -> Selector/1
  Memory/1 -> MATLAB Function/1(u_l)
  MATLAB Function/1(u) -> u/1, Memory/1
  MATLAB Function/2(alpha) -> Memory1/1, alpha [rad]/1
  Clock/1 -> Memory2/1, MATLAB Function/4(clock)
  Memory2/1 -> MATLAB Function/5(clock_l)

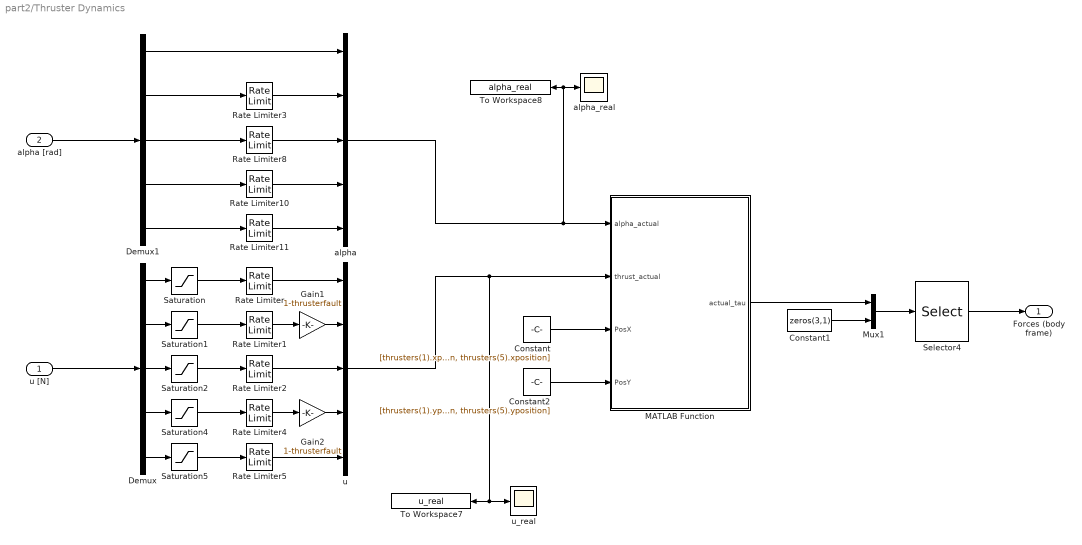
== system part2/Thruster Dynamics ==
  u [N] : Inport
  alpha [rad] : Inport  Port=2
  Constant : Constant  Value=[thrusters(1).xposition, thrusters(2).xposition, thrusters(3).xposition, thrusters(4).xposition, thrusters(5).xposition]
  Constant1 : Constant  Value=zeros(3,1)
  Constant2 : Constant  Value=[thrusters(1).yposition, thrusters(2).yposition, thrusters(3).yposition, thrusters(4).yposition, thrusters(5).yposition]
  Demux : Demux  Outputs=5
  Demux1 : Demux  Outputs=5
  Gain1 : Gain  Gain=1-thrusterfault
  Gain2 : Gain  Gain=1-thrusterfault
  MATLAB Function : MATLAB Function  TreatAsAtomicUnit=on
  Mux1 : Mux  Inputs=2
  Rate Limiter : RateLimiter  RisingSlewLimit=thrusters(1).rate  FallingSlewLimit=-thrusters(1).rate  SampleTimeMode=inherited
  Rate Limiter1 : RateLimiter  RisingSlewLimit=thrusters(2).rate  FallingSlewLimit=-thrusters(2).rate  SampleTimeMode=inherited
  Rate Limiter10 : RateLimiter  RisingSlewLimit=thrusters(4).rotationspeed  FallingSlewLimit=-thrusters(4).rotationspeed  SampleTimeMode=inherited
  Rate Limiter11 : RateLimiter  RisingSlewLimit=thrusters(5).rotationspeed  FallingSlewLimit=-thrusters(5).rotationspeed  SampleTimeMode=inherited
  Rate Limiter2 : RateLimiter  RisingSlewLimit=thrusters(3).rate  FallingSlewLimit=-thrusters(3).rate  SampleTimeMode=inherited
  Rate Limiter3 : RateLimiter  RisingSlewLimit=thrusters(3).rotationspeed  FallingSlewLimit=-thrusters(3).rotationspeed  SampleTimeMode=inherited
  Rate Limiter4 : RateLimiter  RisingSlewLimit=thrusters(4).rate  FallingSlewLimit=-thrusters(4).rate  SampleTimeMode=inherited
  Rate Limiter5 : RateLimiter  RisingSlewLimit=thrusters(5).rate  FallingSlewLimit=-thrusters(5).rate  SampleTimeMode=inherited
  Rate Limiter8 : RateLimiter  RisingSlewLimit=thrusters(3).rotationspeed  FallingSlewLimit=-thrusters(3).rotationspeed  SampleTimeMode=inherited
  Saturation : Saturate  UpperLimit=thrusters(1).thrust  LowerLimit=-thrusters(1).thrust
  Saturation1 : Saturate  UpperLimit=thrusters(2).thrust  LowerLimit=-thrusters(2).thrust
  Saturation2 : Saturate  UpperLimit=thrusters(3).thrust  LowerLimit=-thrusters(3).thrust
  Saturation4 : Saturate  UpperLimit=thrusters(4).thrust  LowerLimit=-thrusters(4).thrust
  Saturation5 : Saturate  UpperLimit=thrusters(5).thrust  LowerLimit=-thrusters(5).thrust
  Selector4 : Selector  InputPortWidth=6  IndexOptions=Index vector (dialog)  Indices=[1 2 4 5 6 3]  OutputSizes=1
  To Workspace7 : ToWorkspace  VariableName=u_real  SaveFormat=Timeseries  SampleTime=-1
  To Workspace8 : ToWorkspace  VariableName=alpha_real  SaveFormat=Timeseries  SampleTime=-1
  alpha : Mux  Inputs=5
  alpha_real : Scope
  u : Mux  Inputs=5
  u_real : Scope
  "Forces (body frame) " : Outport  VectorParamsAs1DForOutWhenUnconnected=off
  wires:
  Rate Limiter2/1 -> u/3
  Saturation/1 -> Rate Limiter/1
  Mux1/1 -> Selector4/1
  Constant1/1 -> Mux1/2
  Saturation4/1 -> Rate Limiter4/1
  Demux/2 -> Saturation1/1
  Saturation1/1 -> Rate Limiter1/1
  Demux/1 -> Saturation/1
  Demux/3 -> Saturation2/1
  Saturation2/1 -> Rate Limiter2/1
  Selector4/1 -> "Forces (body frame) "/1
  Gain1/1 -> u/2
  Rate Limiter1/1 -> Gain1/1
  Rate Limiter/1 -> u/1
  Rate Limiter4/1 -> Gain2/1
  Saturation5/1 -> Rate Limiter5/1
  Rate Limiter8/1 -> alpha/3
  u [N]/1 -> Demux/1
  alpha [rad]/1 -> Demux1/1
  Constant/1 -> MATLAB Function/3(PosX)
  Constant2/1 -> MATLAB Function/4(PosY)
  MATLAB Function/1(actual_tau) -> Mux1/1
  Demux1/3 -> Rate Limiter8/1
  Rate Limiter10/1 -> alpha/4
  Demux1/4 -> Rate Limiter10/1
  Demux1/5 -> Rate Limiter11/1
  Rate Limiter11/1 -> alpha/5
  Demux1/2 -> Rate Limiter3/1
  Demux1/1 -> alpha/1
  Gain2/1 -> u/4
  Demux/4 -> Saturation4/1
  Demux/5 -> Saturation5/1
  Rate Limiter5/1 -> u/5
  Rate Limiter3/1 -> alpha/2
  u/1 -> u_real/1, To Workspace7/1, MATLAB Function/2(thrust_actual)
  alpha/1 -> alpha_real/1, To Workspace8/1, MATLAB Function/1(alpha_actual)

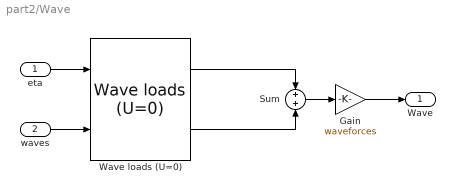
== system part2/Wave ==
  eta : Inport
  waves : Inport  Port=2
  Gain : Gain  Gain=waveforces
  Sum : Sum
  Wave loads (U=0) : marine_hydro/Hydro Library/Wave loads (U=0)  SystemSampleTime=-1  Latency=0  AutoFrameSizeCalculation=off
      settings: SourceProductName=MSS Hydro
  Wave : Outport  VectorParamsAs1DForOutWhenUnconnected=off
  wires:
  eta/1 -> Wave loads (U=0)/1
  waves/1 -> Wave loads (U=0)/2
  Sum/1 -> Gain/1
  Wave loads (U=0)/1 -> Sum/1
  Wave loads (U=0)/2 -> Sum/2
  Gain/1 -> Wave/1

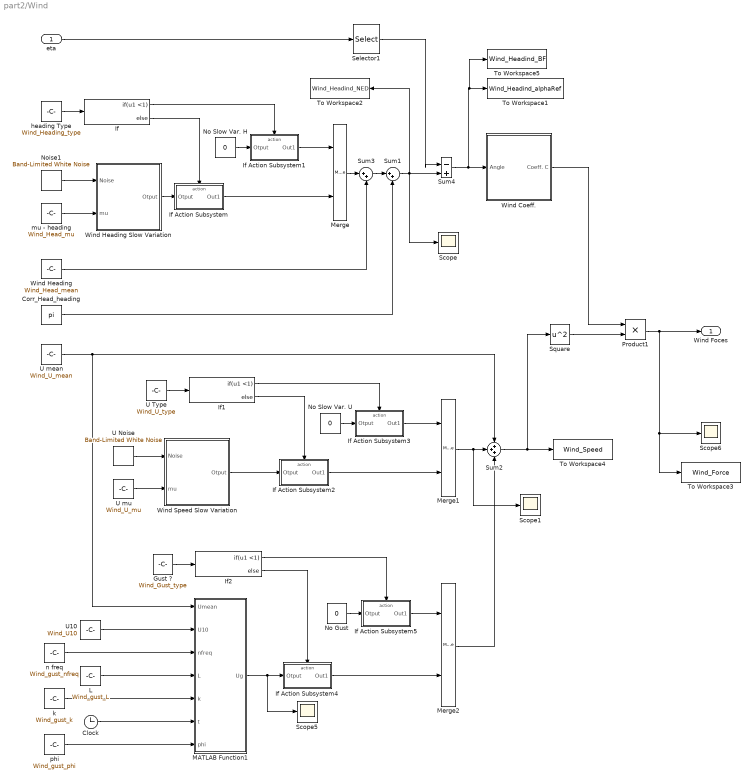
== system part2/Wind ==
  eta : Inport
  Clock : Clock
  Corr_Head_heading : Constant  Value=pi
  Gust ? : Constant  Value=Wind_Gust_type
  If : If  IfExpression=u1 <1
  If Action Subsystem : Subsystem  TreatAsAtomicUnit=on
  If Action Subsystem1 : Subsystem  TreatAsAtomicUnit=on
  If Action Subsystem2 : Subsystem  TreatAsAtomicUnit=on
  If Action Subsystem3 : Subsystem  TreatAsAtomicUnit=on
  If Action Subsystem4 : Subsystem  TreatAsAtomicUnit=on
  If Action Subsystem5 : Subsystem  TreatAsAtomicUnit=on
  If1 : If  IfExpression=u1 <1
  If2 : If  IfExpression=u1 <1
  L : Constant  Value=Wind_gust_L
  MATLAB Function1 : MATLAB Function  TreatAsAtomicUnit=on
  Merge : Merge
  Merge1 : Merge
  Merge2 : Merge
  No Gust : Constant  Value=0
  No Slow Var. H : Constant  Value=0
  No Slow Var. U : Constant  Value=0
  Noise1 : simulink/Sources/Band-Limited White Noise  Cov=Wind_Head_noise_power  Ts=Wind_Head_Sample_time  seed=Wind_Head_Seed
  Product1 : Product
  Scope{,1,5..6} (4 alike) : Scope
  Selector1 : Selector  InputPortWidth=6  IndexOptions=Index vector (dialog)  Indices=[6]  OutputSizes=1
  Square : Math  Operator=square  SaturateOnIntegerOverflow=on
  Sum1 : Sum  Inputs=|++
  Sum2 : Sum  Inputs=+++
  Sum3 : Sum  Inputs=|++
  Sum4 : Sum  Inputs=|-+
  To Workspace1 : ToWorkspace  VariableName=Wind_Headind_alphaRef  SaveFormat=Timeseries  SampleTime=-1
  To Workspace2 : ToWorkspace  VariableName=Wind_Headind_NED  SaveFormat=Timeseries  SampleTime=-1
  To Workspace3 : ToWorkspace  VariableName=Wind_Force  SaveFormat=Timeseries  SampleTime=-1
  To Workspace4 : ToWorkspace  VariableName=Wind_Speed  SaveFormat=Timeseries  SampleTime=-1
  To Workspace5 : ToWorkspace  VariableName=Wind_Headind_BF  SaveFormat=Timeseries  SampleTime=-1
  U Noise : simulink/Sources/Band-Limited White Noise  Cov=Wind_U_noise_power  Ts=Wind_U_Sample_time  seed=Wind_U_Seed
  U Type : Constant  Value=Wind_U_type
  U mean : Constant  Value=Wind_U_mean
  "U mu " : Constant  Value=Wind_U_mu
  U10 : Constant  Value=Wind_U10
  Wind Coeff. : Subsystem
  Wind Heading : Constant  Value=Wind_Head_mean
  Wind Heading Slow Variation : Subsystem
  Wind Speed Slow Variation : Subsystem
  heading Type : Constant  Value=Wind_Heading_type
  k : Constant  Value=Wind_gust_k
  mu - heading : Constant  Value=Wind_Head_mu
  n freq : Constant  Value=Wind_gust_nfreq
  phi : Constant  Value=Wind_gust_phi
  Wind Foces : Outport  VectorParamsAs1DForOutWhenUnconnected=off
  wires:
  If Action Subsystem3/1(Out1) -> Merge1/1
  No Gust/1 -> If Action Subsystem5/1(Otput)
  n freq/1 -> MATLAB Function1/3(nfreq)
  If2/1 -> If Action Subsystem5/Action
  MATLAB Function1/1(Ug) -> Scope5/1, If Action Subsystem4/1(Otput)
  Sum1/1 -> To Workspace2/1, Sum4/2, Scope/1
  If Action Subsystem1/1(Out1) -> Merge/1
  If Action Subsystem/1(Out1) -> Merge/2
  If2/2 -> If Action Subsystem4/Action
  If/1 -> If Action Subsystem1/Action
  Product1/1 -> Scope6/1, To Workspace3/1, Wind Foces/1
  phi/1 -> MATLAB Function1/7(phi)
  Square/1 -> Product1/2
  U Type/1 -> If1/1
  Gust ?/1 -> If2/1
  Wind Coeff./1(Coeff. C) -> Product1/1
  Merge2/1 -> Sum2/3
  U mean/1 -> MATLAB Function1/1(Umean), Sum2/1
  "U mu "/1 -> Wind Speed Slow Variation/2(mu)
  If/2 -> If Action Subsystem/Action
  Sum2/1 -> To Workspace4/1, Square/1
  Wind Speed Slow Variation/1(Otput) -> If Action Subsystem2/1(Otput)
  Selector1/1 -> Sum4/1
  Merge/1 -> Sum3/1
  If1/2 -> If Action Subsystem2/Action
  Sum3/1 -> Sum1/1
  If1/1 -> If Action Subsystem3/Action
  No Slow Var. U/1 -> If Action Subsystem3/1(Otput)
  heading Type/1 -> If/1
  Merge1/1 -> Scope1/1, Sum2/2
  No Slow Var. H/1 -> If Action Subsystem1/1(Otput)
  If Action Subsystem4/1(Out1) -> Merge2/2
  U10/1 -> MATLAB Function1/2(U10)
  k/1 -> MATLAB Function1/5(k)
  L/1 -> MATLAB Function1/4(L)
  Sum4/1 -> To Workspace5/1, To Workspace1/1, Wind Coeff./1(Angle)
  U Noise/1 -> Wind Speed Slow Variation/1(Noise)
  mu - heading/1 -> Wind Heading Slow Variation/2(mu)
  Clock/1 -> MATLAB Function1/6(t)
  If Action Subsystem2/1(Out1) -> Merge1/2
  If Action Subsystem5/1(Out1) -> Merge2/1
  eta/1 -> Selector1/1
  Wind Heading/1 -> Sum3/2
  Wind Heading Slow Variation/1(Otput) -> If Action Subsystem/1(Otput)
  Corr_Head_heading/1 -> Sum1/2
  Noise1/1 -> Wind Heading Slow Variation/1(Noise)

== system part2/Current (North - East)/If Action Subsystem ==
  Otput : Inport
  Action Port : ActionPort  ActionPortLabel=else
  Out1 : Outport
  wires:
  Otput/1 -> Out1/1

== system part2/Current (North - East)/If Action Subsystem1 ==
  Otput : Inport
  Action Port : ActionPort  ActionPortLabel=if(u1 <1)
  Out1 : Outport
  wires:
  Otput/1 -> Out1/1

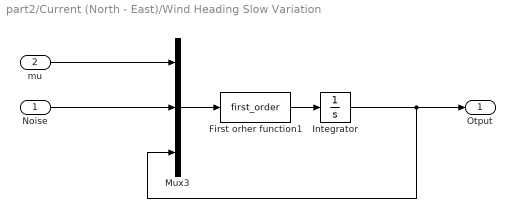
== system part2/Current (North - East)/Wind Heading Slow Variation ==
  Noise : Inport
  mu : Inport  Port=2
  First orher function1 : MATLABFcn  MATLABFcn=first_order
  Integrator : Integrator
  Mux3 : Mux  Inputs=3
  Otput : Outport
  wires:
  First orher function1/1 -> Integrator/1
  Mux3/1 -> First orher function1/1
  mu/1 -> Mux3/1
  Integrator/1 -> Otput/1, Mux3/3
  Noise/1 -> Mux3/2

== system part2/Wind/If Action Subsystem ==
  Otput : Inport
  Action Port : ActionPort  ActionPortLabel=else
  Out1 : Outport
  wires:
  Otput/1 -> Out1/1

== system part2/Wind/If Action Subsystem1 ==
  Otput : Inport
  Action Port : ActionPort  ActionPortLabel=if(u1 <1)
  Out1 : Outport
  wires:
  Otput/1 -> Out1/1

== system part2/Wind/If Action Subsystem2 ==
  Otput : Inport
  Action Port : ActionPort  ActionPortLabel=else
  Out1 : Outport
  wires:
  Otput/1 -> Out1/1

== system part2/Wind/If Action Subsystem3 ==
  Otput : Inport
  Action Port : ActionPort  ActionPortLabel=if(u1 <1)
  Out1 : Outport
  wires:
  Otput/1 -> Out1/1

== system part2/Wind/If Action Subsystem4 ==
  Otput : Inport
  Action Port : ActionPort  ActionPortLabel=else
  Out1 : Outport
  wires:
  Otput/1 -> Out1/1

== system part2/Wind/If Action Subsystem5 ==
  Otput : Inport
  Action Port : ActionPort  ActionPortLabel=if(u1 <1)
  Out1 : Outport
  wires:
  Otput/1 -> Out1/1

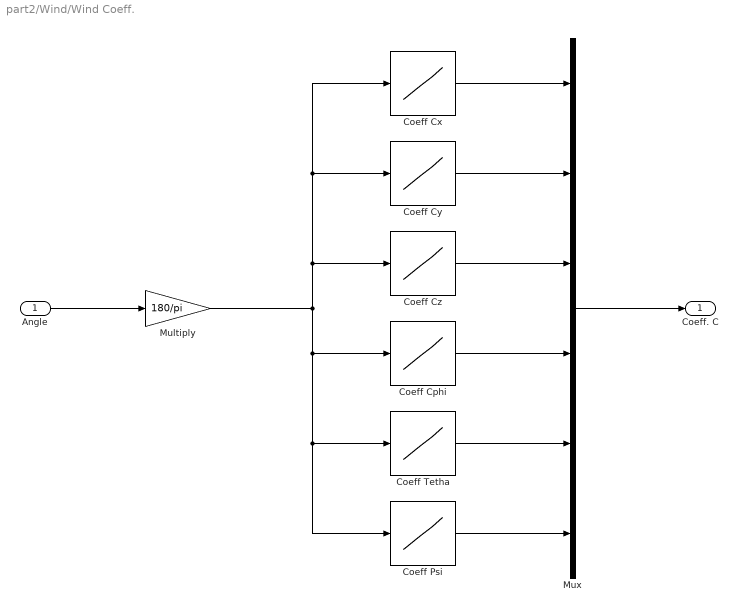
== system part2/Wind/Wind Coeff. ==
  Angle : Inport
  Coeff Cphi : Lookup_n-D  NumberOfTableDimensions=1  BreakpointsForDimension1=|  Table=|  InternalRulePriority=Speed  RndMeth=Simplest  InputSameDT=on
      BreakpointsForDimension1=|
      | [0 , 10 , 20 , 30 , 40 , 50 , 60 , 70 , 80 , 90 , 100 , 110 , 120 , 130 , 140 , 150 , 160 , 170 , 180 , 190 , 200 , 210 , 220 , 230 , 240 , 250 , 260 , 270 , 280 , 290 , 300 , 310 , 320 , 330 , 340 , 350 , 360 
      | ]
      Table=|
      | [0 , 275.994 , 612.99 , 1074.42 , 1437.39 , 1712.25 , 1782.45 , 1678.32 , 1694.25 , 1755.045 , 1739.835 , 1771.92 , 1838.97 , 1769.67 , 1246.185 , 902.88 , 561.195 , 253.215 , 0 , -253.215 , -561.195 , -902.88 , -1246.185 , -1769.67 , -1838.97 , -1771.92 , -1739.835 , -1755.045 , -1694.25 , -1678.32 , -1782.45 , -1712.25 , -1437.39 , -1074.42 , -612.99 , -275.994 , 0
      | ]
  Coeff Cx : Lookup_n-D  NumberOfTableDimensions=1  BreakpointsForDimension1=|  Table=|  InternalRulePriority=Speed  RndMeth=Simplest  InputSameDT=on
      BreakpointsForDimension1=|
      | [0 , 10 , 20 , 30 , 40 , 50 , 60 , 70 , 80 , 90 , 100 , 110 , 120 , 130 , 140 , 150 , 160 , 170 , 180 , 190 , 200 , 210 , 220 , 230 , 240 , 250 , 260 , 270 , 280 , 290 , 300 , 310 , 320 , 330 , 340 , 350 , 360 
      | ]
      Table=|
      | [298.04 , 318.23 , 268.96 , 178.84 , 161.23 , 116.16 , 49.64 , 19.77 , 0.36 , -4.47 , -29.85 , -73.54 , -130.2 , -203.22 , -247.96 , -242.39 , -235.81 , -217.84 , -249.86 , -217.84 , -235.81 , -242.39 , -247.96 , -203.22 , -130.2 , -73.54 , -29.85 , -4.47 , 0.36 , 19.77 , 49.64 , 116.16 , 161.23 , 178.84 , 268.96 , 318.23 , 298.04
      | ]
  Coeff Cy : Lookup_n-D  NumberOfTableDimensions=1  BreakpointsForDimension1=|  Table=[0 , 61.332 , 136.22 , 238.76 , 319.42 , 380.5 , 396.1 , 372.96 , 376.5 , 390.01 , 386.63 , 393.76 , 408.66 , 393.26 , 276.93 , 200.64 , 124.71 , 56.27 , 0 , -56.27 , -124.71 , -200.64 , -276.93 , -393.26 , -408.66 , -393.76 , -386.63 , -390.01 , -376.5 , -372.96 , -396.1 , -380.5 , -319.42 , -238.76 , -136.22 , -61.332 , 0 ]  InternalRulePriority=Speed  RndMeth=Simplest  InputSameDT=on
      | [0 , 10 , 20 , 30 , 40 , 50 , 60 , 70 , 80 , 90 , 100 , 110 , 120 , 130 , 140 , 150 , 160 , 170 , 180 , 190 , 200 , 210 , 220 , 230 , 240 , 250 , 260 , 270 , 280 , 290 , 300 , 310 , 320 , 330 , 340 , 350 , 360 
      | ]
  Coeff Cz : Lookup_n-D  NumberOfTableDimensions=1  BreakpointsForDimension1=|  Table=|  InternalRulePriority=Speed  RndMeth=Simplest  InputSameDT=on
      BreakpointsForDimension1=|
      | [0 , 10 , 20 , 30 , 40 , 50 , 60 , 70 , 80 , 90 , 100 , 110 , 120 , 130 , 140 , 150 , 160 , 170 , 180 , 190 , 200 , 210 , 220 , 230 , 240 , 250 , 260 , 270 , 280 , 290 , 300 , 310 , 320 , 330 , 340 , 350 , 360
      | ]
      Table=|
      | [0 , 0 , 0 , 0 , 0 , 0 , 0 , 0 , 0 , 0 , 0 , 0 , 0 , 0 , 0 , 0 , 0 , 0 , 0 , 0 , 0 , 0 , 0 , 0 , 0 , 0 , 0 , 0 , 0 , 0 , 0 , 0 , 0 , 0 , 0 , 0 , 0
      | ]
  Coeff Psi : Lookup_n-D  NumberOfTableDimensions=1  BreakpointsForDimension1=|  Table=|  InternalRulePriority=Speed  RndMeth=Simplest  InputSameDT=on
      BreakpointsForDimension1=|
      | [0 , 10 , 20 , 30 , 40 , 50 , 60 , 70 , 80 , 90 , 100 , 110 , 120 , 130 , 140 , 150 , 160 , 170 , 180 , 190 , 200 , 210 , 220 , 230 , 240 , 250 , 260 , 270 , 280 , 290 , 300 , 310 , 320 , 330 , 340 , 350 , 360 
      | ]
      Table=|
      | [0 , 551.1 , 661.56 , 451.37 , 212.51 , -23.578 , 1168.3 , 2376.3 , 3511.9 , 4610.4 , 4769.5 , 5921.9 , 6542.8 , 6805.2 , 6751.5 , 6190.1 , 3758.8 , 1905.6 , 0 , -1905.6 , -3758.8 , -6190.1 , -6751.5 , -6805.2 , -6542.8 , -5921.9 , -4769.5 , -4610.4 , -3511.9 , -2376.3 , -1168.3 , 23.578 , -212.51 , -451.37 , -661.56 , -551.1 , 0
      | ]
  Coeff Tetha : Lookup_n-D  NumberOfTableDimensions=1  BreakpointsForDimension1=|  Table=|  InternalRulePriority=Speed  RndMeth=Simplest  InputSameDT=on
      BreakpointsForDimension1=|
      | [0 , 10 , 20 , 30 , 40 , 50 , 60 , 70 , 80 , 90 , 100 , 110 , 120 , 130 , 140 , 150 , 160 , 170 , 180 , 190 , 200 , 210 , 220 , 230 , 240 , 250 , 260 , 270 , 280 , 290 , 300 , 310 , 320 , 330 , 340 , 350 , 360
      | ]
      Table=|
      | [-2355.232759 , -2514.732759 , -2125.37069 , -1413.215517 , -1274.103448 , -917.9310345 , -392.2448276 , -156.2474138 , -2.883896552 , 35.30431034 , 235.9215517 , 581.112931 , 1028.87931 , 1605.905172 , 1959.422414 , 1915.422414 , 1863.456897 , 1721.405172 , 1974.5 , 1721.405172 , 1863.456897 , 1915.422414 , 1959.422414 , 1605.905172 , 1028.87931 , 581.112931 , 235.9215517 , 35.30431034 , -2.883896552 , -156.2474138 , -392.2448276 , -917.9310345 , -1274.103448 , -1413.215517 , -2125.37069 , -2514.732759 , -2355.232759
      | ]
  Multiply : Gain  Gain=180/pi
  Mux : Mux  Inputs=6
  Coeff. C : Outport
  wires:
  Angle/1 -> Multiply/1
  Coeff Psi/1 -> Mux/6
  Coeff Cx/1 -> Mux/1
  Coeff Cy/1 -> Mux/2
  Coeff Cz/1 -> Mux/3
  Coeff Cphi/1 -> Mux/4
  Coeff Tetha/1 -> Mux/5
  Mux/1 -> Coeff. C/1
  Multiply/1 -> Coeff Psi/1, Coeff Tetha/1, Coeff Cphi/1, Coeff Cx/1, Coeff Cy/1, Coeff Cz/1

== system part2/Wind/Wind Heading Slow Variation ==
  Noise : Inport
  mu : Inport  Port=2
  First orher function1 : MATLABFcn  MATLABFcn=first_order
  Integrator : Integrator
  Mux3 : Mux  Inputs=3
  Otput : Outport
  wires:
  First orher function1/1 -> Integrator/1
  Mux3/1 -> First orher function1/1
  mu/1 -> Mux3/1
  Integrator/1 -> Otput/1, Mux3/3
  Noise/1 -> Mux3/2

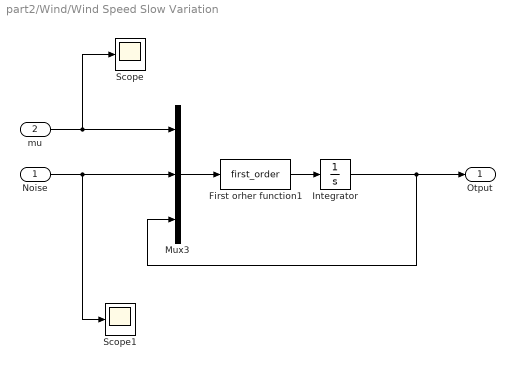
== system part2/Wind/Wind Speed Slow Variation ==
  Noise : Inport
  mu : Inport  Port=2
  First orher function1 : MATLABFcn  MATLABFcn=first_order
  Integrator : Integrator
  Mux3 : Mux  Inputs=3
  Scope : Scope
  Scope1 : Scope
  Otput : Outport
  wires:
  First orher function1/1 -> Integrator/1
  Mux3/1 -> First orher function1/1
  mu/1 -> Scope/1, Mux3/1
  Integrator/1 -> Otput/1, Mux3/3
  Noise/1 -> Scope1/1, Mux3/2

== matlab function part2/Wind/MATLAB Function1 ==
  data: Umean input; U10 input; nfreq input; L input; k input; t input; Ug output; phi input
function Ug   = windGust(Umean,U10,nfreq,L,k,t,phi)

%     nfreq = 100;
%     L = 1800;
%     k = 0.0026;
    
%     Umean = input(1);
%     U10 = input(2);
%     nfreq = input(3);
%     L = input(4);
%     k = input(5);
%     t = input(6);

    Ug = 0;
    
    freq = zeros(nfreq,1);
    S = zeros(nfreq,1);
    
    for i = 1:nfreq
        freq(i,1) = 0.01 + (i-1)/(nfreq-1) * 0.99;
        ftilde = L*freq(i,1)/Umean;
        S(i,1) = (4*k*L*U10) / ((2+ftilde^2)^(5/6));
    end

    for i = 1:nfreq
        Ug = Ug + sqrt(2*S(i,1)*(freq(2,1)-freq(1,1))) * cos(2*pi*freq(i,1)*t + phi(i,1));
    end


end

== matlab function part2/Observer  Kalman Filter/MATLAB Function ==
  data: p_bar output; p_bar input; x_bar input; h input; x_bar output; y input; eta_hat output; nu_hat output; tau_est input; A input; B input; D input; E input; H input; invT input; invM input; Q input; R input
function [p_bar,x_bar, eta_hat,nu_hat]=EKF(p_bar,x_bar,h,y,tau_est,A,B,D,E,H,invT,invM,Q,R)

% kalman gain
K= p_bar *H'*inv(H*p_bar*H'+R);

% error covariance
p_hat=(eye(15)-K*H)*p_bar*(eye(15)-K*H)'+K*R*K';

% estimate with meassuremtn
x_hat=x_bar+K*(y-H*x_bar);

%rotation matrix
rot=rotz(x_hat(9)*180/pi);

drotz=[-sin(x_hat(9)) -cos(x_hat(9)) 0;
    cos(x_hat(9)) -sin(x_hat(9)) 0;
    0 0 0];

%control plant model
f=[A, zeros(6,3), zeros(6,3), zeros(6,3);
    zeros(3,6), zeros(3), zeros(3), rot;
    zeros(3,6), zeros(3), -invT, zeros(3);
    zeros(3,6), zeros(3), invM*rot', -invM*D];

df=[A, zeros(6,9);
    zeros(3,6), zeros(3,2), drotz*x_hat(13:15), zeros(3), rot;
    zeros(3,9), -invT, zeros(3);
    zeros(3,6), zeros(3,2), invM*drotz*x_hat(10:12), invM*rot',-invM*D];

%Kalman state matrices
Phi=eye(15)+h*df;
Gamma=h*E;

%Predictor
x_bar = x_hat+h*(f*x_hat+B*tau_est);
p_bar = Phi*p_hat*Phi'+Gamma*Q*Gamma';

eta_hat = x_hat(7:9);
nu_hat = x_hat(13:15);
end
